simulink model "poles"  (R2018a)
settings: Solver=VariableStepAuto  StartTime=0.0  StopTime=10.0  RelTol=1e-3
values from neighbouring files (symbols this model uses):
  B = 20e3    (= 20000)    [LAB2.m]
  j = 600e3    (= 600000)    [LAB2.m]
  k = 2000    [LAB2.m]
settings Model: Creator=Ahmed Eldokmak  LastModifiedBy=Ahmed Eldokmak

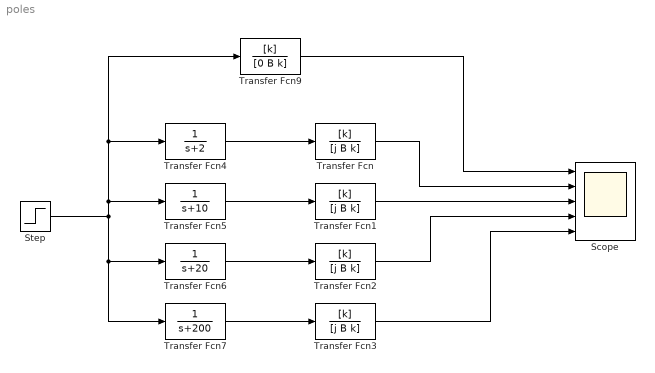
== system poles ==
  Scope : Scope  NumInputPorts=5
  Step : Step  SampleTime=0
  Transfer Fcn{,1..3} (4 alike) : TransferFcn  Numerator=[k]  Denominator=[j B k]
  Transfer Fcn4 : TransferFcn  Denominator=[1 2]
  Transfer Fcn5 : TransferFcn  Denominator=[1 10]
  Transfer Fcn6 : TransferFcn  Denominator=[1 20]
  Transfer Fcn7 : TransferFcn  Denominator=[1 200]
  Transfer Fcn9 : TransferFcn  Numerator=[k]  Denominator=[0 B k]
  wires:
  Transfer Fcn4/1 -> Transfer Fcn/1
  Transfer Fcn5/1 -> Transfer Fcn1/1
  Transfer Fcn6/1 -> Transfer Fcn2/1
  Transfer Fcn7/1 -> Transfer Fcn3/1
  Step/1 -> Transfer Fcn5/1, Transfer Fcn9/1, Transfer Fcn4/1, Transfer Fcn7/1, Transfer Fcn6/1
  Transfer Fcn9/1 -> Scope/1
  Transfer Fcn/1 -> Scope/2
  Transfer Fcn1/1 -> Scope/3
  Transfer Fcn2/1 -> Scope/4
  Transfer Fcn3/1 -> Scope/5
